simulink model "SetResetWaitOut"  (Simulink 5.0)
settings: Solver=ode45  StartTime=0.0  StopTime=10.0  RelTol=1e-3
settings Model: Creator=scaife  LastModifiedBy=scaife  ExtModeAutoUpdateStatusClock=off

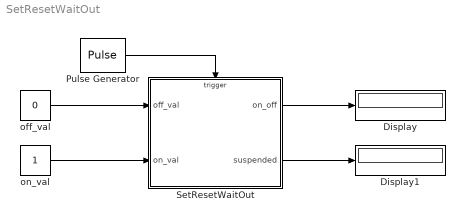
== system SetResetWaitOut ==
  Display : Display
  Display1 : Display
  Pulse Generator : DiscretePulseGenerator  PulseType=Time based  PulseWidth=50
  SetResetWaitOut : Stateflow chart
  off_val : Constant  Value=0
  on_val : Constant
  wires:
  off_val/1 -> SetResetWaitOut/1(off_val)
  on_val/1 -> SetResetWaitOut/2(on_val)
  SetResetWaitOut/1(on_off) -> Display/1
  SetResetWaitOut/2(suspended) -> Display1/1
  Pulse Generator/1 -> SetResetWaitOut/Trigger

== stateflow chart SetResetWaitOut ==
  state Wait/
    en: suspended=1;
    ex: suspended=0;
  state Off/
    en: on_off=0;
  state On/
    en: on_off=1;
  (default) -> Off
  Wait -> Off : Clear
  Off -> Wait : Suspend
  Off -> On : Set
  On -> Off : Reset
  On -> Wait : Suspend
  data: on_off output int32; suspended output uint32; off_val input int32; on_val input int32
  events: Clear input EITHER_EDGE_EVENT; Suspend input EITHER_EDGE_EVENT; Set input EITHER_EDGE_EVENT; Reset input EITHER_EDGE_EVENT
